simulink model "Interleaved_boost_control"  (R2020a)
settings: Solver=VariableStepAuto  StartTime=0.0  StopTime=1  RelTol=1e-3  EnableMultiTasking=on
libraries: powerlib x17, simulink x1
settings Model: Creator=sunil  LastModifiedBy=sunil
settings DataIOCC: ReturnWorkspaceOutputs=off
settings OptimizationCC: LifeSpan=inf
settings DebuggingCC: SFUnexpectedBacktrackingDiag=warning  SFNoUnconditionalDefaultTransitionDiag=warning  ArithmeticOperatorsInVariantConditions=warning
settings SFSimCC: SimUseLocalCustomCode=off  CustomCodeUndefinedFunction=UseInterfaceOnly
settings RTWCC: RTWUseLocalCustomCode=off
settings CodeAppCC: StateflowObjectComments=on
settings GRTTargetCC: TargetLangStandard=C89/C90 (ANSI)
settings ConfigComp: CovMetricSettings=dw  CovHtmlReporting=on  CovSaveCumulativeToWorkspaceVar=on  CovSaveSingleToWorkspaceVar=on  CovExternalEMLEnable=off
settings SimscapeCC: SimscapeNormalizeSystem=off

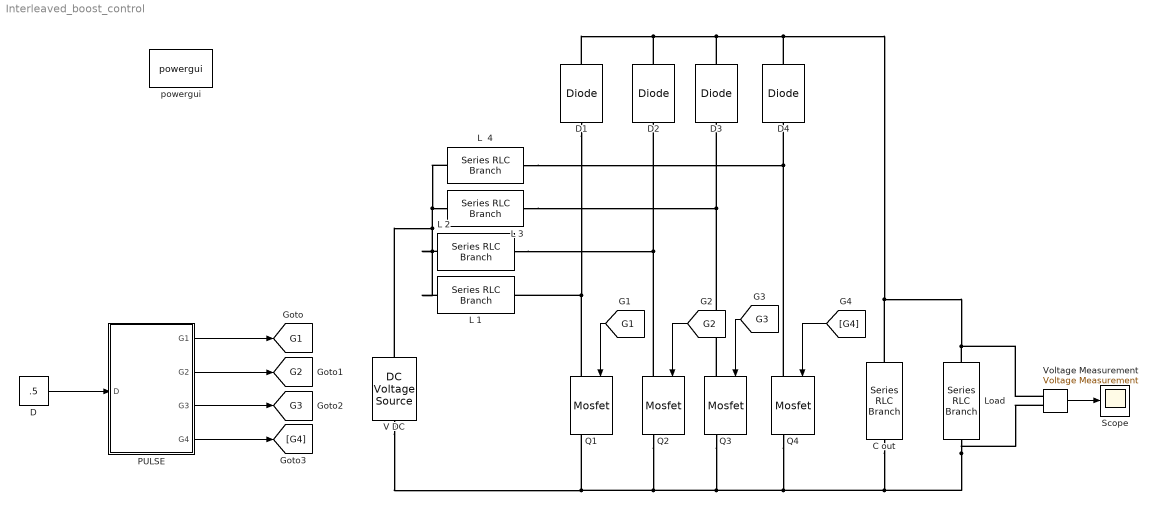
== system Interleaved_boost_control ==
  "  Load  " : powerlib/Elements/Series RLC Branch  LConnTagsString=__new0  RConnTagsString=__new0  BranchType=R  Resistance=180  Inductance=400e-6  SetiL0=off  InitialCurrent=0  Capacitance=1e-6  Setx0=off  InitialVoltage=0  Measurements=None
  "  V DC" : powerlib/Electrical Sources/DC Voltage Source  Amplitude=200  Measurements=None
  " Voltage Measurement" : powerlib/Measurements/Voltage Measurement  PhasorSimulation=off  OutputType=Complex  PSBequivalent=0
  C out : powerlib/Elements/Series RLC Branch  LConnTagsString=__new0  RConnTagsString=__new0  BranchType=C  Resistance=1  Inductance=400e-6  SetiL0=off  InitialCurrent=0  Capacitance=195e-6  Setx0=off  InitialVoltage=0  Measurements=None
  D : Constant  Value=.5
  D{1..4} (4 alike) : powerlib/Power Electronics/Diode  Ron=0.001  Lon=0  Vf=0.8  IC=0  UseSnubber=off  Rs=500  Cs=250e-9  Measurements=off
  L  4 : powerlib/Elements/Series RLC Branch  LConnTagsString=__new0  RConnTagsString=__new0  BranchType=L  Resistance=1  Inductance=100e-6  SetiL0=off  InitialCurrent=0  Capacitance=1e-6  Setx0=off  InitialVoltage=0  Measurements=None
  L 1 : powerlib/Elements/Series RLC Branch  LConnTagsString=__new0  RConnTagsString=__new0  BranchType=L  Resistance=1  Inductance=100e-6  SetiL0=off  InitialCurrent=0  Capacitance=1e-6  Setx0=off  InitialVoltage=0  Measurements=None
  L 2 : powerlib/Elements/Series RLC Branch  LConnTagsString=__new0  RConnTagsString=__new0  BranchType=L  Resistance=1  Inductance=100e-6  SetiL0=off  InitialCurrent=0  Capacitance=1e-6  Setx0=off  InitialVoltage=0  Measurements=None
  L 3 : powerlib/Elements/Series RLC Branch  LConnTagsString=__new0  RConnTagsString=__new0  BranchType=L  Resistance=1  Inductance=100e-6  SetiL0=off  InitialCurrent=0  Capacitance=1e-6  Setx0=off  InitialVoltage=0  Measurements=None
  PULSE : Subsystem
  Q1 : powerlib/Power Electronics/Mosfet  Ron=0.1  Lon=0  Rd=0.01  Vfd=0  IC=0  Rs=1e5  Cs=inf  Measurements=on
  "Q2 " : powerlib/Power Electronics/Mosfet  Ron=0.1  Lon=0  Rd=0.01  Vfd=0  IC=0  Rs=1e5  Cs=inf  Measurements=on
  "Q3  " : powerlib/Power Electronics/Mosfet  Ron=0.1  Lon=0  Rd=0.01  Vfd=0  IC=0  Rs=1e5  Cs=inf  Measurements=on
  "Q4 " : powerlib/Power Electronics/Mosfet  Ron=0.1  Lon=0  Rd=0.01  Vfd=0  IC=0  Rs=1e5  Cs=inf  Measurements=on
  Scope : Scope
  powergui : powerlib/powergui  Priority=1  SimulationMode=Discrete  SampleTime=5e-6  frequency=60  Iterations=50  frequencyindice=0  Pbase=100e6  ErrMax=1e-4  UnitsV=kV  UnitsW=MW  buscounter=0  FunctionMessages=off  echomessages=off  EnableUseOfTLC=off  CurrentSourceSwitches=off  DisableSnubberDevices=off  DisableRonSwitches=off  DisableVfSwitches=off  DisplayEquations=off  AutomaticDiscreteSolvers=off  SolverType=Tustin/Backward Euler (TBE)  Interpol=off  ExternalGateDelay=off  methode=off  Ts=10  x0status=blocks  SPID=off  SwTol=0  HookPort=off  NonlinearTolerance=1e-4  nMaxIteration=100  ContinueOnMaxIteration=off  RestoreLinks=warning  ResistiveCurrentMeasurement=off  Frange=[0:2:500]  Ylog=off  Xlog=on  ShowGrid=off  save=off  variable=ZData  structure=0  ZoomFFT=off  StartTime=0.0  cycles=1  DisplayStyle=1  fundamental=60  FreqAxis=off  MaxFrequency=1000  frequencyindicesteady=1  RmsSteady=1  display=off
  tag scope: G1=global, G2=global, G3=global
  wires:
  " Voltage Measurement"/1 -> Scope/1
  [G3] -> "Q3  "/1
  D/1 -> PULSE/1(D)
  [G1] -> Q1/1
  PULSE/1(G1) -> [G1]
  PULSE/2(G2) -> [G2]
  PULSE/3(G3) -> [G3]
  PULSE/4(G4) -> [G4]
  [G4] -> "Q4 "/1
  [G2] -> "Q2 "/1
  connections:
  Q1/LConn1 -- D1/LConn1 -- L 1/RConn1
  "  V DC"/LConn1 -- " Voltage Measurement"/LConn2 -- "  Load  "/RConn1 -- C out/RConn1 -- "Q4 "/RConn1 -- "Q3  "/RConn1 -- "Q2 "/RConn1 -- Q1/RConn1
  C out/LConn1 -- D1/RConn1 -- D2/RConn1 -- D3/RConn1 -- D4/RConn1 -- " Voltage Measurement"/LConn1 -- "  Load  "/LConn1
  "Q2 "/LConn1 -- D2/LConn1 -- L 2/RConn1
  "Q3  "/LConn1 -- D3/LConn1 -- L 3/RConn1
  "Q4 "/LConn1 -- D4/LConn1 -- L  4/RConn1
  L  4/LConn1 -- L 1/LConn1 -- L 2/LConn1 -- "  V DC"/RConn1 -- L 3/LConn1

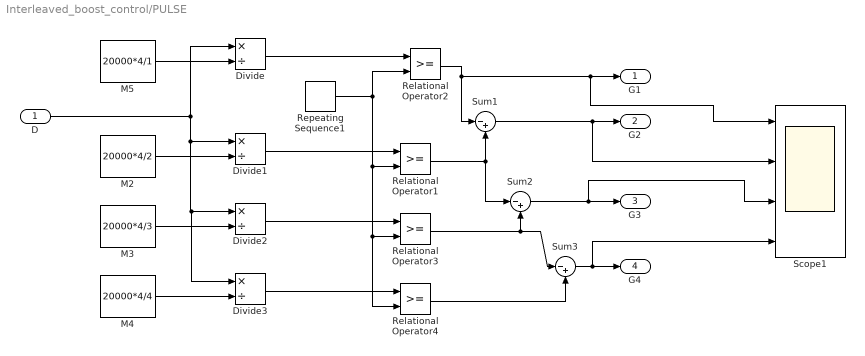
== system Interleaved_boost_control/PULSE ==
  D : Inport
  Divide{,1..3} (4 alike) : Product  Inputs=*/
  M2 : Constant  Value=20000*4/2
  M3 : Constant  Value=20000*4/3
  M4 : Constant  Value=20000*4/4
  M5 : Constant  Value=20000*4/1
  Relational Operator{1..4} (4 alike) : RelationalOperator  OutDataTypeStr=boolean  RndMeth=Nearest
  Repeating Sequence1 : simulink/Sources/Repeating Sequence  rep_seq_t=[0 1/20000]  rep_seq_y=[0 1/20000]
  Scope1 : Scope  NumInputPorts=4
  Sum1 : Sum  Inputs=|-+
  Sum2 : Sum  Inputs=|-+
  Sum3 : Sum  Inputs=|-+
  G1 : Outport
  G2 : Outport  Port=2
  G3 : Outport  Port=3
  G4 : Outport  Port=4
  wires:
  Sum1/1 -> Scope1/2, G2/1
  D/1 -> Divide/1, Divide3/1, Divide2/1, Divide1/1
  Relational Operator2/1 -> Sum1/1, Scope1/1, G1/1
  Repeating Sequence1/1 -> Relational Operator4/2, Relational Operator3/2, Relational Operator1/2, Relational Operator2/2
  Divide1/1 -> Relational Operator1/1
  Divide2/1 -> Relational Operator3/1
  Divide3/1 -> Relational Operator4/1
  M5/1 -> Divide/2
  Divide/1 -> Relational Operator2/1
  Relational Operator1/1 -> Sum1/2, Sum2/1
  M2/1 -> Divide1/2
  M3/1 -> Divide2/2
  M4/1 -> Divide3/2
  Relational Operator3/1 -> Sum3/1, Sum2/2
  Sum2/1 -> Scope1/3, G3/1
  Sum3/1 -> Scope1/4, G4/1
  Relational Operator4/1 -> Sum3/2
